simulink model "SecRwRtStFtrstCtrl"  (R2018b)
settings: Solver=FixedStepDiscrete  StartTime=0.0  StopTime=10.0  FixedStep=0.01  RelTol=1e-3
undefined symbols (not defined in the file or in its folder): KeSMSuMdMotFinshdTm_Val, KeSMSuMdRetryTm1_Val, KeSMSuModeReqDurgTm_Val, KeSMSwSecRwRtStFtrstEnTrigBitMask_Val
libraries: StCtrlLib x1
settings Model: Creator=sn2xws  LastModifiedBy=sn2xws
settings DataIOCC: SaveFormat=StructureWithTime
settings OptimizationCC: DefaultParameterBehavior=Inlined  EnhancedBackFolding=on  PassReuseOutputArgsAs=Individual arguments  ZeroExternalMemoryAtStartup=off  ZeroInternalMemoryAtStartup=off  OptimizeBlockOrder=speed  DifferentSizesBufferReuse=on  OptimizationCustomize=off
settings DebuggingCC: ParameterTunabilityLossMsg=error
settings ModelReferenceCC: ModelReferenceNumInstancesAllowed=Single
settings SFSimCC: MATLABDynamicMemAlloc=off
settings RTWCC: SystemTargetFile=autosar.tlc  GenCodeOnly=on  TemplateMakefile=ert_default_tmf  Description=AUTOSAR  GenerateReport=on  IncludeHyperlinkInReport=on  LaunchReport=on  GenerateTraceInfo=on  GenerateTraceReport=on  GenerateTraceReportSl=on  GenerateTraceReportSf=on  GenerateTraceReportEml=on
settings CodeAppCC: ForceParamTrailComments=on  IgnoreCustomStorageClasses=off  OperatorAnnotations=on  SimulinkDataObjDesc=on  SFDataObjDesc=on  InsertBlockDesc=on
settings STFCustomTargetCC: TargetLangStandard=C99 (ISO)  MultiwordLength=256  ParMdlRefBuildCompliant=on  CompOptLevelCompliant=on  IncludeMdlTerminateFcn=off  CombineOutputUpdateFcns=on  SuppressErrorStatus=on  ERTCustomFileBanners=on  SupportNonFinite=off  SupportComplex=off  SupportContinuousTime=off  SupportNonInlinedSFcns=off  RemoveResetFunc=on  MATLABClassNameForMDSCustomization=Simulink.SoftwareTarget.ERTCustomization  AutosarCompliant=on  UseToolchainInfoCompliant=on  LookupTableObjectStructAxisOrder=2,1,3,4,...  LUTObjectStructOrderEvenSpacing=Size,Table,Breakpoints  SystemTargetFile=autosar.tlc
settings ERTTargetCC: TargetLangStandard=C99 (ISO)  ConcurrentExecutionCompliant=off  IncludeMdlTerminateFcn=off  SuppressErrorStatus=on  SupportNonFinite=off  SupportComplex=off  ModelStepFunctionPrototypeControlCompliant=off  CPPClassGenCompliant=off  AutosarCompliant=on  LookupTableObjectStructAxisOrder=2,1,3,4,...  LUTObjectStructOrderEvenSpacing=Size,Table,Breakpoints  InlinedParameterPlacement=NonHierarchical  ERTCustomFileTemplate=example_file_process.tlc  ERTFilePackagingFormat=Compact

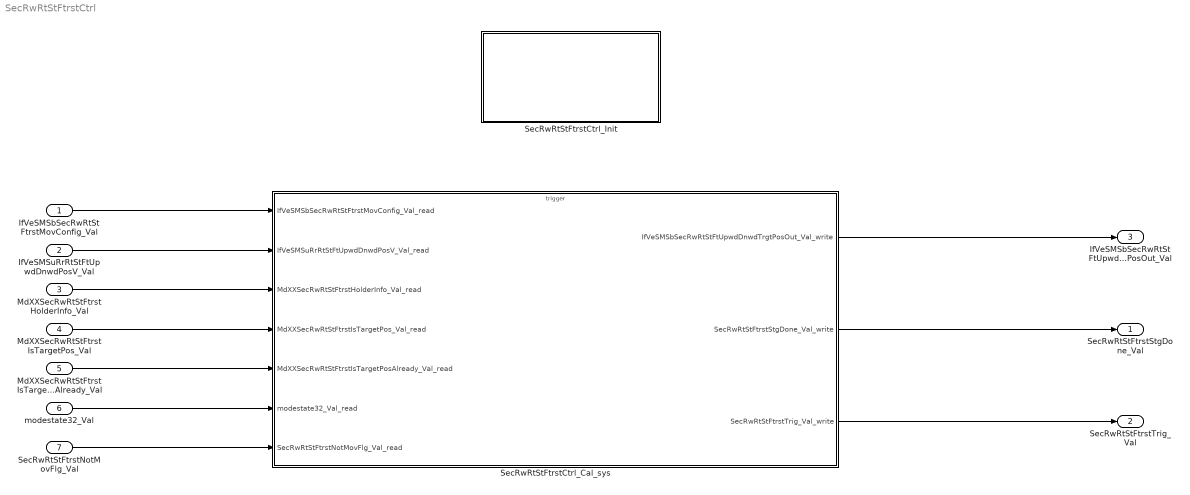
== system SecRwRtStFtrstCtrl ==
  IfVeSMSbSecRwRtStFtrstMovConfig_Val : Inport  OutDataTypeStr=boolean  PortDimensions=1
  IfVeSMSuRrRtStFtUpwdDnwdPosV_Val : Inport  Port=2  OutDataTypeStr=boolean  PortDimensions=1
  MdXXSecRwRtStFtrstHolderInfo_Val : Inport  Port=3  OutDataTypeStr=uint32  PortDimensions=1
  MdXXSecRwRtStFtrstIsTargetPos_Val : Inport  Port=4  OutDataTypeStr=uint32  PortDimensions=1
  MdXXSecRwRtStFtrstIsTargetPosAlready_Val : Inport  Port=5  OutDataTypeStr=uint32  PortDimensions=1
  modestate32_Val : Inport  Port=6  OutDataTypeStr=uint32  PortDimensions=1
  SecRwRtStFtrstNotMovFlg_Val : Inport  Port=7  OutDataTypeStr=boolean  PortDimensions=1
  SecRwRtStFtrstCtrl_Cal_sys : Subsystem
  SecRwRtStFtrstCtrl_Init : Subsystem
  SecRwRtStFtrstStgDone_Val : Outport  OutDataTypeStr=boolean  PortDimensions=1
  SecRwRtStFtrstTrig_Val : Outport  Port=2  OutDataTypeStr=boolean  PortDimensions=1
  IfVeSMSbSecRwRtStFtUpwdDnwdTrgtPosOut_Val : Outport  Port=3  OutDataTypeStr=boolean  PortDimensions=1
  wires:
  SecRwRtStFtrstCtrl_Cal_sys/1(IfVeSMSbSecRwRtStFtUpwdDnwdTrgtPosOut_Val_write) -> IfVeSMSbSecRwRtStFtUpwdDnwdTrgtPosOut_Val/1
  SecRwRtStFtrstCtrl_Cal_sys/2(SecRwRtStFtrstStgDone_Val_write) -> SecRwRtStFtrstStgDone_Val/1
  SecRwRtStFtrstCtrl_Cal_sys/3(SecRwRtStFtrstTrig_Val_write) -> SecRwRtStFtrstTrig_Val/1
  IfVeSMSbSecRwRtStFtrstMovConfig_Val/1 -> SecRwRtStFtrstCtrl_Cal_sys/1(IfVeSMSbSecRwRtStFtrstMovConfig_Val_read)
  IfVeSMSuRrRtStFtUpwdDnwdPosV_Val/1 -> SecRwRtStFtrstCtrl_Cal_sys/2(IfVeSMSuRrRtStFtUpwdDnwdPosV_Val_read)
  MdXXSecRwRtStFtrstHolderInfo_Val/1 -> SecRwRtStFtrstCtrl_Cal_sys/3(MdXXSecRwRtStFtrstHolderInfo_Val_read)
  MdXXSecRwRtStFtrstIsTargetPos_Val/1 -> SecRwRtStFtrstCtrl_Cal_sys/4(MdXXSecRwRtStFtrstIsTargetPos_Val_read)
  MdXXSecRwRtStFtrstIsTargetPosAlready_Val/1 -> SecRwRtStFtrstCtrl_Cal_sys/5(MdXXSecRwRtStFtrstIsTargetPosAlready_Val_read)
  modestate32_Val/1 -> SecRwRtStFtrstCtrl_Cal_sys/6(modestate32_Val_read)
  SecRwRtStFtrstNotMovFlg_Val/1 -> SecRwRtStFtrstCtrl_Cal_sys/7(SecRwRtStFtrstNotMovFlg_Val_read)

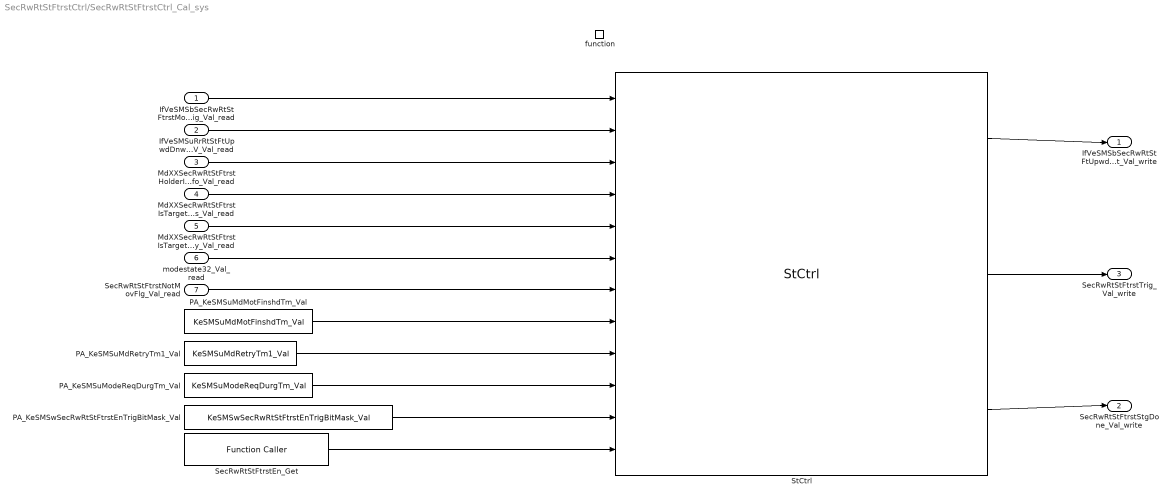
== system SecRwRtStFtrstCtrl/SecRwRtStFtrstCtrl_Cal_sys ==
  IfVeSMSbSecRwRtStFtrstMovConfig_Val_read : Inport
  IfVeSMSuRrRtStFtUpwdDnwdPosV_Val_read : Inport  Port=2
  MdXXSecRwRtStFtrstHolderInfo_Val_read : Inport  Port=3
  MdXXSecRwRtStFtrstIsTargetPos_Val_read : Inport  Port=4
  MdXXSecRwRtStFtrstIsTargetPosAlready_Val_read : Inport  Port=5
  modestate32_Val_read : Inport  Port=6
  SecRwRtStFtrstNotMovFlg_Val_read : Inport  Port=7
  function : TriggerPort  TriggerType=function-call  IsSimulinkFunction=on  FunctionName=SecRwRtStFtrstCtrl_Cal  VariantControl=(inherit)
  PA_KeSMSuMdMotFinshdTm_Val : Constant  Value=KeSMSuMdMotFinshdTm_Val
  PA_KeSMSuMdRetryTm1_Val : Constant  Value=KeSMSuMdRetryTm1_Val
  PA_KeSMSuModeReqDurgTm_Val : Constant  Value=KeSMSuModeReqDurgTm_Val
  PA_KeSMSwSecRwRtStFtrstEnTrigBitMask_Val : Constant  Value=KeSMSwSecRwRtStFtrstEnTrigBitMask_Val
  SecRwRtStFtrstEn_Get : FunctionCaller  FunctionPrototype=data = SecRwRtStFtrstEn_Get()  OutputArgumentSpecifications=uint32(1)
  StCtrl : StCtrlLib/StCtrl  SystemSampleTime=-1
  IfVeSMSbSecRwRtStFtUpwdDnwdTrgtPosOut_Val_write : Outport
      settings: EnsureOutportIsVirtual=on
  SecRwRtStFtrstStgDone_Val_write : Outport  Port=2
      settings: EnsureOutportIsVirtual=on
  SecRwRtStFtrstTrig_Val_write : Outport  Port=3
      settings: EnsureOutportIsVirtual=on
  wires:
  StCtrl/1 -> IfVeSMSbSecRwRtStFtUpwdDnwdTrgtPosOut_Val_write/1
  PA_KeSMSwSecRwRtStFtrstEnTrigBitMask_Val/1 -> StCtrl/11
  SecRwRtStFtrstEn_Get/1 -> StCtrl/12
  PA_KeSMSuMdMotFinshdTm_Val/1 -> StCtrl/8
  PA_KeSMSuModeReqDurgTm_Val/1 -> StCtrl/10
  PA_KeSMSuMdRetryTm1_Val/1 -> StCtrl/9
  IfVeSMSbSecRwRtStFtrstMovConfig_Val_read/1 -> StCtrl/1
  IfVeSMSuRrRtStFtUpwdDnwdPosV_Val_read/1 -> StCtrl/2
  MdXXSecRwRtStFtrstHolderInfo_Val_read/1 -> StCtrl/3
  MdXXSecRwRtStFtrstIsTargetPos_Val_read/1 -> StCtrl/4
  MdXXSecRwRtStFtrstIsTargetPosAlready_Val_read/1 -> StCtrl/5
  modestate32_Val_read/1 -> StCtrl/6
  SecRwRtStFtrstNotMovFlg_Val_read/1 -> StCtrl/7
  StCtrl/2 -> SecRwRtStFtrstTrig_Val_write/1
  StCtrl/3 -> SecRwRtStFtrstStgDone_Val_write/1

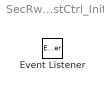
== system SecRwRtStFtrstCtrl/SecRwRtStFtrstCtrl_Init ==
  Event Listener : EventListener  EventName=reset
